simulink model "Modele_LQR_3DOF"  (R2019b)
settings: Solver=VariableStepAuto  StartTime=0.0  StopTime=20  FixedStep=0.1  RelTol=1e-3
undefined symbols (not defined in the file): Amatrix, B, Bmatrix, Fx1, Fx2, Fx3, Fx4, Fx5, Fx6, Fx7, Fx8, Fy1, Fy2, Fy3, Fy4, Fy5, Fy6, Fy7, Fy8, Fz1, Fz2, Fz3, Fz4, Fz5, Fz6, Fz7, Fz8, I_x, I_y, I_z, lx1, lx2, lx3, lx4, lx5, lx6, lx7, lx8, ly1, ly2, ly3, ly4, ly5, ly6, ly7, ly8, lz1, lz2, lz3, lz4, lz5, lz6, lz7, lz8, m, Q, R, W, X0, x_rb ... (+5)
libraries: simulink x12, robotlib x7, dspinverses x1
(part 1 of 2)
settings Model: Creator=ASUQTR  LastModifiedBy=coteba
settings SolverCC: ZeroCrossAlgorithm=Adaptive
settings DebuggingCC: IgnoredZcDiagnostic=none

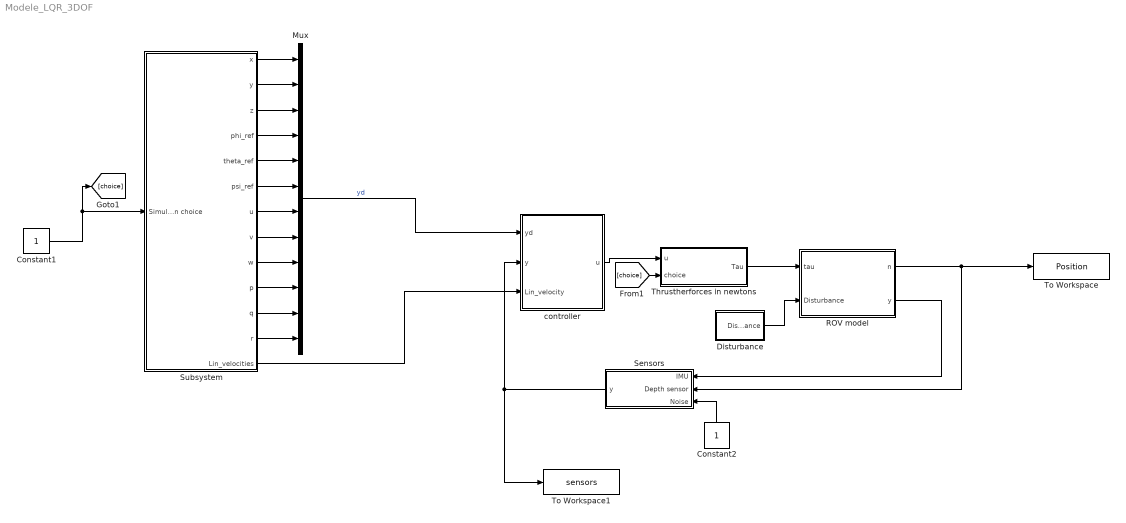
== system Modele_LQR_3DOF ==
  Constant1 : Constant
  Constant2 : Constant
  Disturbance : Subsystem
  Mux : Mux  Inputs=12
  ROV model : Subsystem
  Sensors : Subsystem
  Subsystem : Subsystem
  Thrustherforces in newtons : Subsystem
  To Workspace : ToWorkspace  VariableName=Position  SaveFormat=Structure With Time  SampleTime=-1
  To Workspace1 : ToWorkspace  VariableName=sensors  SaveFormat=Structure With Time  SampleTime=-1
  controller : Subsystem
  wires:
  Mux/1 -> controller/1(yd)  "yd"
  Disturbance/1(Disturbance) -> ROV model/2(Disturbance)
  ROV model/1(n) -> To Workspace/1, Sensors/2(Depth sensor)
  Thrustherforces in newtons/1(Tau) -> ROV model/1(tau)
  controller/1(u) -> Thrustherforces in newtons/1(u)
  Constant1/1 -> [choice], Subsystem/1(Simulation choice)
  Subsystem/13(Lin_velocities) -> controller/3(Lin_velocity)
  [choice] -> Thrustherforces in newtons/2(choice)
  Constant2/1 -> Sensors/3(Noise)
  ROV model/2(y) -> Sensors/1(IMU)
  Subsystem/2("y ") -> Mux/2
  Subsystem/1(x) -> Mux/1
  Subsystem/3("z ") -> Mux/3
  Subsystem/4(phi_ref) -> Mux/4
  Subsystem/5(theta_ref) -> Mux/5
  Subsystem/6(psi_ref) -> Mux/6
  Subsystem/7(u) -> Mux/7
  Subsystem/8(v) -> Mux/8
  Subsystem/9(w) -> Mux/9
  Subsystem/10(p) -> Mux/10
  Subsystem/11(q) -> Mux/11
  Subsystem/12(r) -> Mux/12
  Sensors/1(y) -> To Workspace1/1, controller/2(y)

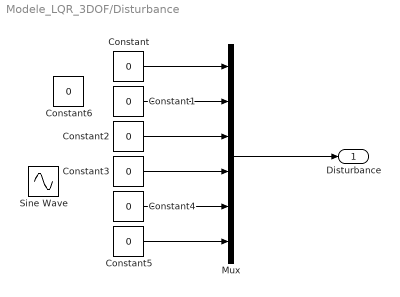
== system Modele_LQR_3DOF/Disturbance ==
  Constant{,1..6} (7 alike) : Constant  Value=0
  Mux : Mux  Inputs=6
  Sine Wave : Sin  Amplitude=0.15  Frequency=10  SampleTime=0
  Disturbance : Outport
  wires:
  Mux/1 -> Disturbance/1
  Constant1/1 -> Mux/2
  Constant2/1 -> Mux/3
  Constant4/1 -> Mux/5
  Constant5/1 -> Mux/6
  Constant/1 -> Mux/1
  Constant3/1 -> Mux/4

== system Modele_LQR_3DOF/ROV model ==
  tau : Inport
  Disturbance : Inport  Port=2
  ROV model : Subsystem
  n : Outport
  y : Outport  Port=2
  wires:
  tau/1 -> ROV model/1(tau)
  Disturbance/1 -> ROV model/2(Disturbance)
  ROV model/2(euler+vitesse_body) -> y/1
  ROV model/1(𝜂) -> n/1

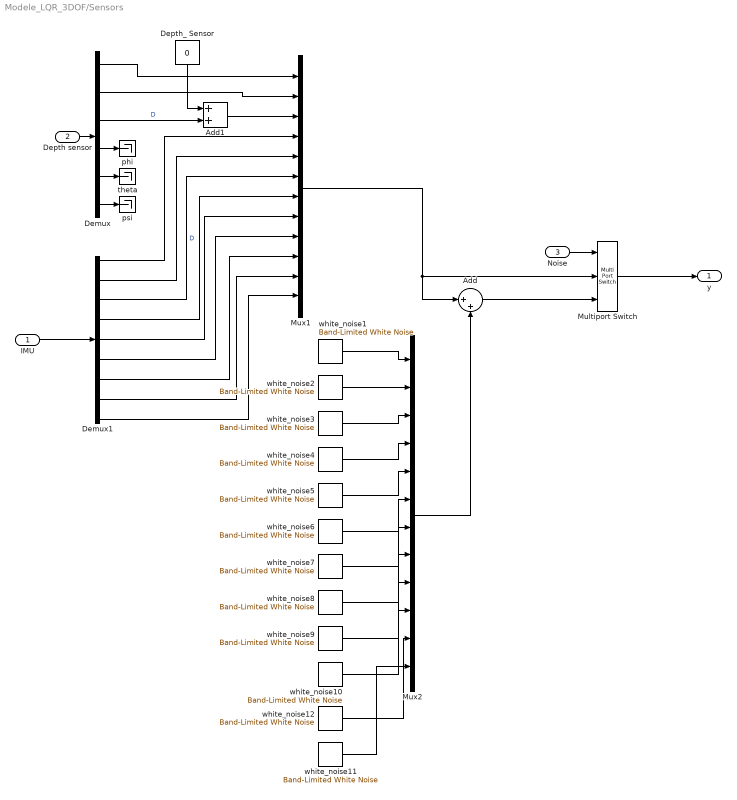
== system Modele_LQR_3DOF/Sensors ==
  IMU : Inport
  Depth sensor : Inport  Port=2
  Noise : Inport  Port=3
  Add : Sum  Inputs=|++
  Add1 : Sum
  Demux : Demux  Outputs=6
  Demux1 : Demux  Outputs=9
  Depth_ Sensor : Constant  Value=0
  Multiport Switch : MultiPortSwitch  Inputs=2
  Mux1 : Mux  Inputs=12
  Mux2 : Mux  Inputs=12
  phi : Terminator
  psi : Terminator
  theta : Terminator
  white_noise1 : simulink/Sources/Band-Limited White Noise  Cov=0.000010  Ts=0.01  seed=[23341]
  white_noise{7..12} (6 alike) : simulink/Sources/Band-Limited White Noise  Cov=0.000010  Ts=0.010000  seed=[8093341]
  white_noise2 : simulink/Sources/Band-Limited White Noise  Cov=0.000010  Ts=0.010000  seed=[23312341]
  white_noise3 : simulink/Sources/Band-Limited White Noise  Cov=0.000010  Ts=0.010000  seed=[2334571]
  white_noise4 : simulink/Sources/Band-Limited White Noise  Cov=0.000010  Ts=0.010000  seed=[21344441]
  white_noise5 : simulink/Sources/Band-Limited White Noise  Cov=0.000010  Ts=0.010000  seed=[3304141]
  white_noise6 : simulink/Sources/Band-Limited White Noise  Cov=0.000010  Ts=0.010000  seed=[903341]
  y : Outport
  wires:
  Multiport Switch/1 -> y/1
  Add/1 -> Multiport Switch/3
  white_noise5/1 -> Mux2/5
  white_noise6/1 -> Mux2/6
  white_noise4/1 -> Mux2/4
  white_noise2/1 -> Mux2/2
  white_noise1/1 -> Mux2/1
  white_noise3/1 -> Mux2/3
  white_noise7/1 -> Mux2/7
  Mux2/1 -> Add/2
  Noise/1 -> Multiport Switch/1
  Mux1/1 -> Multiport Switch/2, Add/1
  white_noise8/1 -> Mux2/8
  white_noise9/1 -> Mux2/9
  white_noise10/1 -> Mux2/10
  Depth sensor/1 -> Demux/1
  Demux/4 -> phi/1
  Demux/5 -> theta/1
  Demux/6 -> psi/1
  Demux/3 -> Add1/2  "D"
  Depth_ Sensor/1 -> Add1/1
  IMU/1 -> Demux1/1
  Add1/1 -> Mux1/3
  Demux/2 -> Mux1/2
  Demux/1 -> Mux1/1
  Demux1/1 -> Mux1/4
  Demux1/2 -> Mux1/5
  Demux1/3 -> Mux1/6  "D"
  Demux1/4 -> Mux1/7
  Demux1/5 -> Mux1/8
  Demux1/6 -> Mux1/9
  Demux1/7 -> Mux1/10
  Demux1/8 -> Mux1/11
  Demux1/9 -> Mux1/12
  white_noise12/1 -> Mux2/11
  white_noise11/1 -> Mux2/12

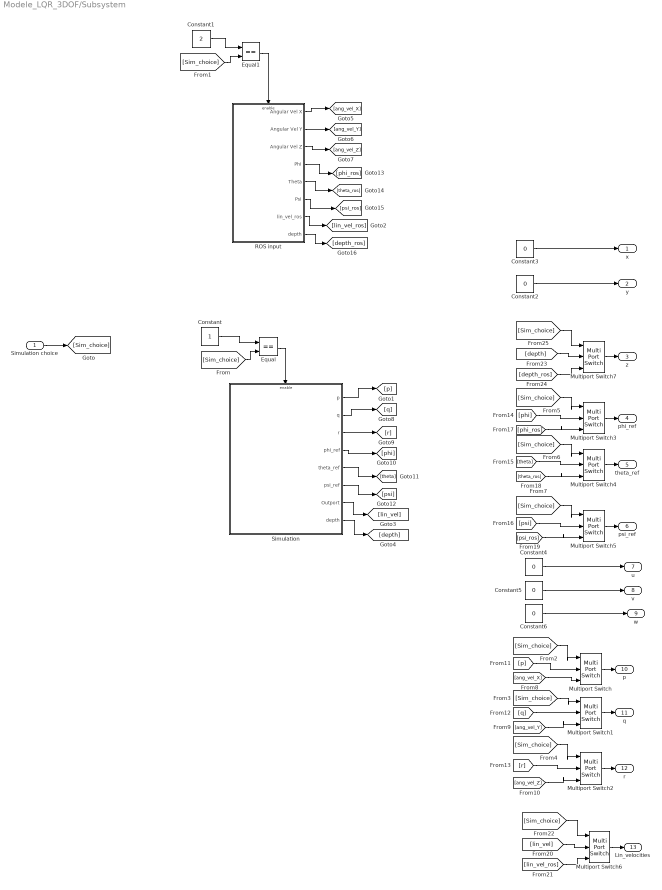
== system Modele_LQR_3DOF/Subsystem ==
  Simulation choice : Inport
  Constant : Constant
  Constant1 : Constant  Value=2
  Constant{2..6} (5 alike) : Constant  Value=0
  Equal : RelationalOperator  Operator===  OutDataTypeStr=boolean  RndMeth=Simplest
  Equal1 : RelationalOperator  Operator===  OutDataTypeStr=boolean  RndMeth=Simplest
  Multiport Switch{,1..7} (8 alike) : MultiPortSwitch  Inputs=2
  ROS input : Subsystem
  Simulation : Subsystem
  x : Outport  VectorParamsAs1DForOutWhenUnconnected=off
  "y " : Outport  Port=2  VectorParamsAs1DForOutWhenUnconnected=off
  "z " : Outport  Port=3  VectorParamsAs1DForOutWhenUnconnected=off
  phi_ref : Outport  Port=4  VectorParamsAs1DForOutWhenUnconnected=off
  theta_ref : Outport  Port=5  VectorParamsAs1DForOutWhenUnconnected=off
  psi_ref : Outport  Port=6  VectorParamsAs1DForOutWhenUnconnected=off
  u : Outport  Port=7  VectorParamsAs1DForOutWhenUnconnected=off
  v : Outport  Port=8  VectorParamsAs1DForOutWhenUnconnected=off
  w : Outport  Port=9  VectorParamsAs1DForOutWhenUnconnected=off
  p : Outport  Port=10  VectorParamsAs1DForOutWhenUnconnected=off
  q : Outport  Port=11  VectorParamsAs1DForOutWhenUnconnected=off
  r : Outport  Port=12  VectorParamsAs1DForOutWhenUnconnected=off
  Lin_velocities : Outport  Port=13  VectorParamsAs1DForOutWhenUnconnected=off
  wires:
  Equal/1 -> Simulation/Enable
  Simulation choice/1 -> [Sim_choice]
  Constant/1 -> Equal/1
  [Sim_choice] -> Equal/2
  Constant1/1 -> Equal1/1
  [Sim_choice] -> Equal1/2
  Equal1/1 -> ROS input/Enable
  Multiport Switch/1 -> p/1
  Multiport Switch1/1 -> q/1
  Multiport Switch2/1 -> r/1
  Multiport Switch3/1 -> phi_ref/1
  Multiport Switch4/1 -> theta_ref/1
  Multiport Switch5/1 -> psi_ref/1
  [Sim_choice] -> Multiport Switch/1
  [Sim_choice] -> Multiport Switch1/1
  [Sim_choice] -> Multiport Switch2/1
  [Sim_choice] -> Multiport Switch3/1
  [Sim_choice] -> Multiport Switch4/1
  [Sim_choice] -> Multiport Switch5/1
  ROS input/1(Angular Vel X) -> [ang_vel_X]
  ROS input/2(Angular Vel Y) -> [ang_vel_Y]
  ROS input/3(Angular Vel Z) -> [ang_vel_Z]
  [ang_vel_X] -> Multiport Switch/3
  [ang_vel_Y] -> Multiport Switch1/3
  [ang_vel_Z] -> Multiport Switch2/3
  Simulation/1(p) -> [p]
  Simulation/2(q) -> [q]
  Simulation/3(r) -> [r]
  Simulation/4(phi_ref) -> [phi]
  Simulation/5(theta_ref) -> [theta]
  Simulation/6(psi_ref) -> [psi]
  [p] -> Multiport Switch/2
  [q] -> Multiport Switch1/2
  [r] -> Multiport Switch2/2
  [phi] -> Multiport Switch3/2
  [theta] -> Multiport Switch4/2
  [psi] -> Multiport Switch5/2
  ROS input/4(Phi) -> [phi_ros]
  ROS input/5(Theta) -> [theta_ros]
  ROS input/6(Psi) -> [psi_ros]
  [phi_ros] -> Multiport Switch3/3
  [theta_ros] -> Multiport Switch4/3
  [psi_ros] -> Multiport Switch5/3
  Simulation/7(Outport) -> [lin_vel]
  [lin_vel_ros] -> Multiport Switch6/3
  [Sim_choice] -> Multiport Switch6/1
  [lin_vel] -> Multiport Switch6/2
  Multiport Switch6/1 -> Lin_velocities/1
  ROS input/7(lin_vel_ros) -> [lin_vel_ros]
  [depth] -> Multiport Switch7/2
  [depth_ros] -> Multiport Switch7/3
  Multiport Switch7/1 -> "z "/1
  [Sim_choice] -> Multiport Switch7/1
  Simulation/8(depth) -> [depth]
  ROS input/8(depth) -> [depth_ros]
  Constant2/1 -> "y "/1
  Constant3/1 -> x/1
  Constant4/1 -> u/1
  Constant5/1 -> v/1
  Constant6/1 -> w/1

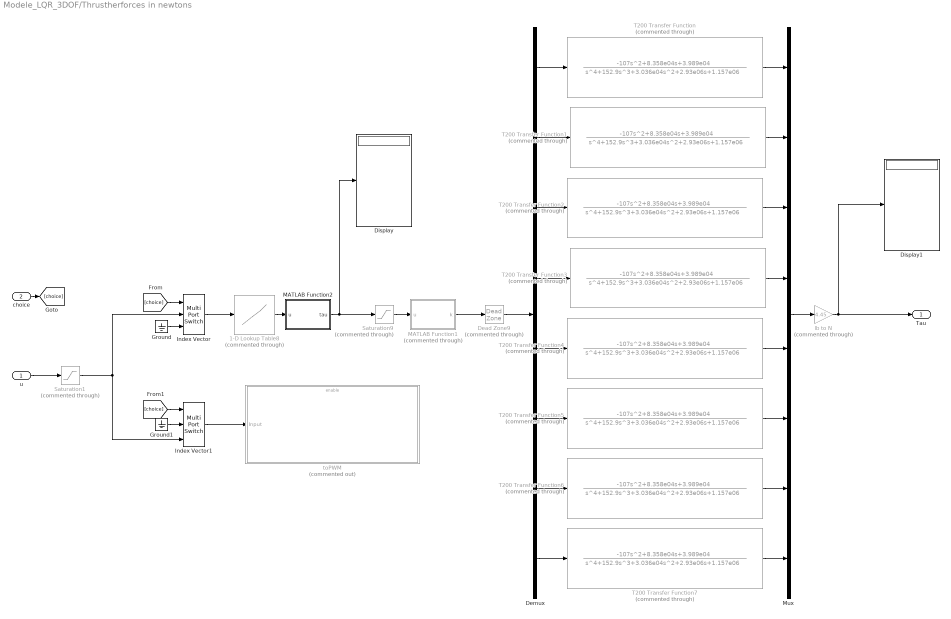
== system Modele_LQR_3DOF/Thrustherforces in newtons ==
  u : Inport
  choice : Inport  Port=2
  1-D Lookup Table8 : Lookup_n-D  Commented=through  NumberOfTableDimensions=1  BreakpointsForDimension1=[-1:0.01:1]  Table=1500 + 400 * ([-1:0.01:1])  InternalRulePriority=Speed  RndMeth=Simplest  InputSameDT=on
  Dead Zone9 : DeadZone  Commented=through  LowerValue=-10  UpperValue=+10  SaturateOnIntegerOverflow=on
  Demux : Demux  Outputs=8
  Display : Display
  Display1 : Display
  Ground : Ground
  Ground1 : Ground
  Index Vector : MultiPortSwitch  DataPortOrder=Specify indices  Inputs=1  DataPortIndices={1,2}
  Index Vector1 : MultiPortSwitch  DataPortOrder=Specify indices  Inputs=2  DataPortIndices={1,2}
  MATLAB Function1 : MATLAB Function  Commented=through  TreatAsAtomicUnit=on
  MATLAB Function2 : MATLAB Function  TreatAsAtomicUnit=on
  Mux : Mux  Inputs=8
  Saturation1 : Saturate  Commented=through  UpperLimit=1  LowerLimit=-1
  Saturation9 : Saturate  Commented=through  UpperLimit=1900  LowerLimit=1100
  T200 Transfer Function{,1..7} (8 alike) : TransferFcn  Commented=through  Numerator="[-107  8.358e04  3.989e04]"  Denominator="[1 152.9  3.036e04  2.93e06  1.157e06]"
  lb to N : Gain  Commented=through  Gain=4.45
  toPWM : Subsystem  Commented=on
  Tau : Outport
  wires:
  u/1 -> Saturation1/1
  Demux/5 -> T200 Transfer Function4/1
  Demux/4 -> T200 Transfer Function3/1
  Demux/2 -> T200 Transfer Function1/1
  1-D Lookup Table8/1 -> MATLAB Function2/1(u)
  Demux/1 -> T200 Transfer Function/1
  Demux/3 -> T200 Transfer Function2/1
  Demux/6 -> T200 Transfer Function5/1
  Demux/7 -> T200 Transfer Function6/1
  Demux/8 -> T200 Transfer Function7/1
  Dead Zone9/1 -> Demux/1
  T200 Transfer Function1/1 -> Mux/2
  T200 Transfer Function3/1 -> Mux/4
  T200 Transfer Function2/1 -> Mux/3
  T200 Transfer Function/1 -> Mux/1
  T200 Transfer Function4/1 -> Mux/5
  T200 Transfer Function5/1 -> Mux/6
  T200 Transfer Function6/1 -> Mux/7
  T200 Transfer Function7/1 -> Mux/8
  Mux/1 -> lb to N/1
  lb to N/1 -> Display1/1, Tau/1
  Index Vector1/1 -> toPWM/1(Input)
  Saturation1/1 -> Index Vector/2, Index Vector1/3
  Ground/1 -> Index Vector/3
  Ground1/1 -> Index Vector1/2
  choice/1 -> [choice]
  [choice] -> Index Vector/1
  [choice] -> Index Vector1/1
  Index Vector/1 -> 1-D Lookup Table8/1
  Saturation9/1 -> MATLAB Function1/1(u)
  MATLAB Function1/1(k) -> Dead Zone9/1
  MATLAB Function2/1(tau) -> Display/1, Saturation9/1

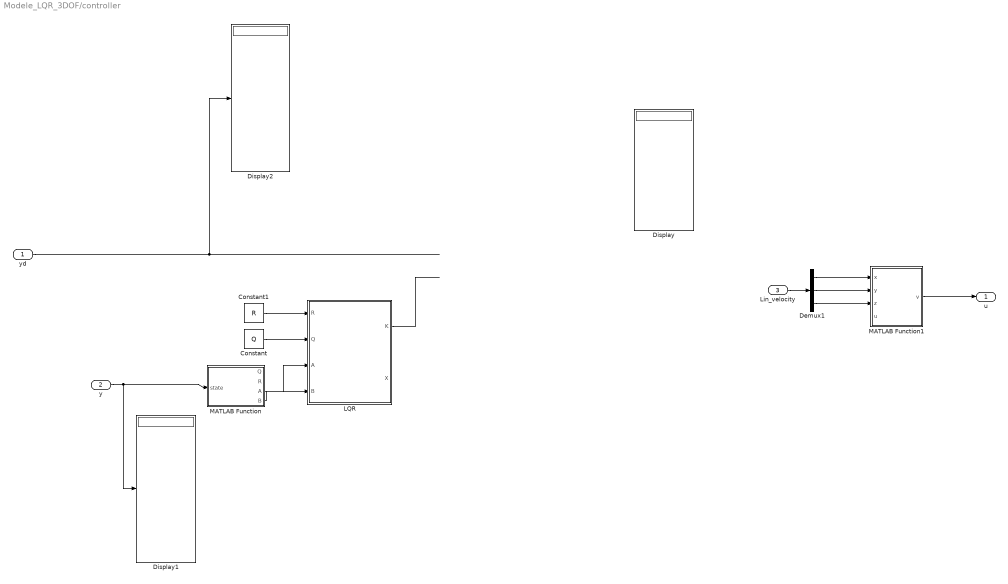
== system Modele_LQR_3DOF/controller ==
  yd : Inport
  y : Inport  Port=2
  Lin_velocity : Inport  Port=3
  Constant : Constant  Value=Q
  Constant1 : Constant  Value=R
  Demux1 : Demux  Outputs=3
  Display : Display
  Display1 : Display
  Display2 : Display
  LQR : Subsystem  Description=|  TreatAsAtomicUnit=on  mask(LQR with Algebric Riccati Equation){A=Amatrix, B=Bmatrix, X0=X0}
      | LQR Block
      | 
      | by Gurkan KAVURAN
      | gurkankavuran@gmail.com
      mask prompts: A "A (System Matrix)"; B "B (System Matrix)"; X0 "Xo (Initial Values of States)"
      mask help:
      | It is easy to optimize Q and R matrices with online process.
      | Please see the help file to define the block parameters.
      mask Help:
      | Parameters Example:
      | 
      | Q = diag([500 1 1 0 1 1] );
      | R = 1*diag([0.01 0.01 0.01 0.01]);
      | X0=[0 0 0 0 0 0;0 0 0 0 0 0;0 0 0 0 0 0;0 0 0 0 0 0;0 0 0 0 0 0;0 0 0 0 0 0];
      | 
      | "Matrix multiply" block is recommended to use in state feedback control mechanism.
      | 
      | 
      | http://www.gurkankavuran.com
      mask Display:
      | disp('LQR')
      | port_label('input', 1, 'R')
      | port_label('input', 2, 'Q')
      | port_label('output', 1, 'K')
      | port_label('output', 2, 'X')
  MATLAB Function : MATLAB Function  TreatAsAtomicUnit=on
  MATLAB Function1 : MATLAB Function  TreatAsAtomicUnit=on
  u : Outport
  wires:
  Constant1/1 -> LQR/1(R)
  Constant/1 -> LQR/2(Q)
  LQR/1(K) -> ?
  ? -> MATLAB Function1/4(u), Display/1
  Lin_velocity/1 -> Demux1/1
  yd/1 -> Display2/1
  MATLAB Function1/1(v) -> u/1
  Demux1/2 -> MATLAB Function1/2(y)
  Demux1/1 -> MATLAB Function1/1(x)
  Demux1/3 -> MATLAB Function1/3(z)
  MATLAB Function/3(A) -> LQR/3(A)
  MATLAB Function/4(B) -> LQR/4("B ")
  y/1 -> Display1/1, MATLAB Function/1(state)

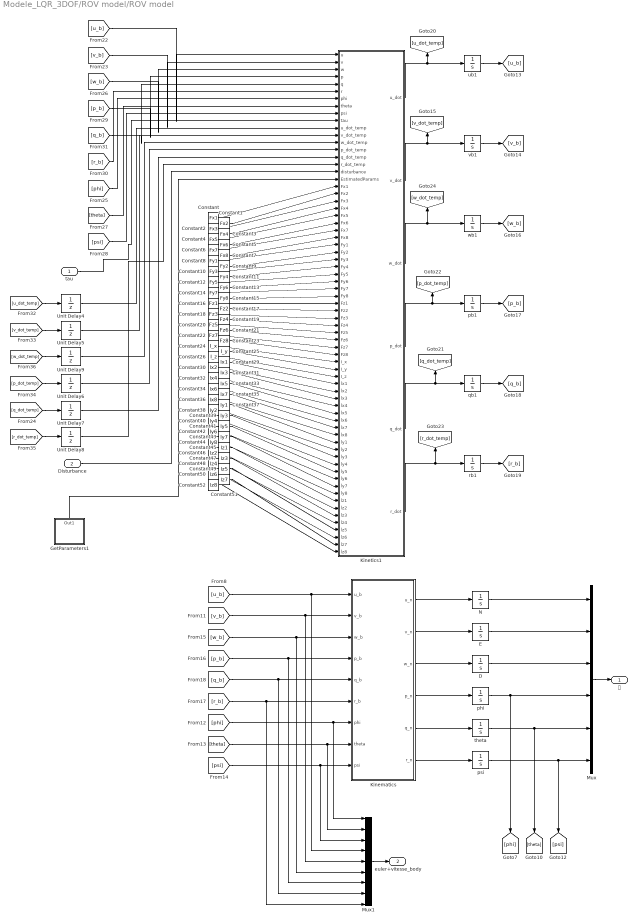
== system Modele_LQR_3DOF/ROV model/ROV model ==
  tau : Inport
  Disturbance : Inport  Port=2
  Constant : Constant  Value=Fx1
  Constant1 : Constant  Value=Fx2
  Constant10 : Constant  Value=Fy3
  Constant11 : Constant  Value=Fy4
  Constant12 : Constant  Value=Fy5
  Constant13 : Constant  Value=Fy6
  Constant14 : Constant  Value=Fy7
  Constant15 : Constant  Value=Fy8
  Constant16 : Constant  Value=Fz1
  Constant17 : Constant  Value=Fz2
  Constant18 : Constant  Value=Fz3
  Constant19 : Constant  Value=Fz4
  Constant2 : Constant  Value=Fx3
  Constant20 : Constant  Value=Fz5
  Constant21 : Constant  Value=Fz6
  Constant22 : Constant  Value=Fz7
  Constant23 : Constant  Value=Fz8
  Constant24 : Constant  Value=I_x
  Constant25 : Constant  Value=I_y
  Constant26 : Constant  Value=I_z
  Constant29 : Constant  Value=lx1
  Constant3 : Constant  Value=Fx4
  Constant30 : Constant  Value=lx2
  Constant31 : Constant  Value=lx3
  Constant32 : Constant  Value=lx4
  Constant33 : Constant  Value=lx5
  Constant34 : Constant  Value=lx6
  Constant35 : Constant  Value=lx7
  Constant36 : Constant  Value=lx8
  Constant37 : Constant  Value=ly1
  Constant38 : Constant  Value=ly2
  Constant39 : Constant  Value=ly3
  Constant4 : Constant  Value=Fx5
  Constant40 : Constant  Value=ly4
  Constant41 : Constant  Value=ly5
  Constant42 : Constant  Value=ly6
  Constant43 : Constant  Value=ly7
  Constant44 : Constant  Value=ly8
  Constant45 : Constant  Value=lz1
  Constant46 : Constant  Value=lz2
  Constant47 : Constant  Value=lz3
  Constant48 : Constant  Value=lz4
  Constant49 : Constant  Value=lz5
  Constant5 : Constant  Value=Fx6
  Constant50 : Constant  Value=lz6
  Constant51 : Constant  Value=lz7
  Constant52 : Constant  Value=lz8
  Constant6 : Constant  Value=Fx7
  Constant7 : Constant  Value=Fx8
  Constant8 : Constant  Value=Fy1
  Constant9 : Constant  Value=Fy2
  D : Integrator  InitialCondition=0.0000001  ContinuousStateAttributes='phi'
  E : Integrator  InitialCondition=0.0000001  ContinuousStateAttributes='phi'
  GetParameters1 : Subsystem
  Kinematics : MATLAB Function  TreatAsAtomicUnit=on
  Kinetics1 : MATLAB Function  TreatAsAtomicUnit=on
  Mux : Mux  Inputs=6
  Mux1 : Mux  Inputs=9
  N : Integrator  InitialCondition=0.0000001  ContinuousStateAttributes='phi'
  Unit Delay{4..9} (6 alike) : UnitDelay  SampleTime=0.01  HasFrameUpgradeWarning=on
  pb1 : Integrator  InitialCondition=0.0000001
  phi : Integrator  InitialCondition=0.0000001  ContinuousStateAttributes='phi'
  psi : Integrator  InitialCondition=0.0000001  ContinuousStateAttributes='psi'
  qb1 : Integrator  InitialCondition=0.0000001
  rb1 : Integrator  InitialCondition=0.0000001
  theta : Integrator  InitialCondition=0.0000001  ContinuousStateAttributes='theta'
  ub1 : Integrator  InitialCondition=0.0000001
  vb1 : Integrator  InitialCondition=0.0000001
  wb1 : Integrator  InitialCondition=0.0000001
  𝜂 : Outport
  euler+vitesse_body : Outport  Port=2
  wires:
  Unit Delay9/1 -> Kinetics1/13(w_dot_temp)
  tau/1 -> Kinetics1/10(tau)
  [phi] -> Kinetics1/7(phi)
  Kinetics1/4(p_dot) -> [p_dot_temp], pb1/1
  [w_dot_temp] -> Unit Delay9/1
  Kinetics1/2(v_dot) -> [v_dot_temp], vb1/1
  [r_b] -> Kinetics1/6(r)
  Kinetics1/6(r_dot) -> rb1/1, [r_dot_temp]
  Unit Delay8/1 -> Kinetics1/16(r_dot_temp)
  [u_b] -> Kinetics1/1(u)
  Unit Delay7/1 -> Kinetics1/15(q_dot_temp)
  rb1/1 -> [r_b]
  Unit Delay6/1 -> Kinetics1/14(p_dot_temp)
  [q_b] -> Kinetics1/5(q)
  [r_dot_temp] -> Unit Delay8/1
  [psi] -> Kinetics1/9(psi)
  [p_dot_temp] -> Unit Delay6/1
  [q_dot_temp] -> Unit Delay7/1
  [p_b] -> Kinetics1/4(p)
  Disturbance/1 -> Kinetics1/17(disturbance)
  Kinetics1/1(u_dot) -> [u_dot_temp], ub1/1
  Unit Delay5/1 -> Kinetics1/12(v_dot_temp)
  [theta] -> Kinetics1/8(theta)
  Kinetics1/5(q_dot) -> qb1/1, [q_dot_temp]
  [v_b] -> Kinetics1/2(v)
  GetParameters1/1(Out1) -> Kinetics1/18(EstimatedParams)
  [w_b] -> Kinetics1/3(w)
  pb1/1 -> [p_b]
  [v_dot_temp] -> Unit Delay5/1
  qb1/1 -> [q_b]
  vb1/1 -> [v_b]
  ub1/1 -> [u_b]
  wb1/1 -> [w_b]
  Kinetics1/3(w_dot) -> [w_dot_temp], wb1/1
  [u_dot_temp] -> Unit Delay4/1
  Unit Delay4/1 -> Kinetics1/11(u_dot_temp)
  [r_b] -> Mux1/9, Kinematics/6(r_b)
  [w_b] -> Mux1/6, Kinematics/3(w_b)
  Kinematics/4(p_n) -> phi/1
  Mux1/1 -> euler+vitesse_body/1
  phi/1 -> Mux/4, [phi]
  Kinematics/5(q_n) -> theta/1
  psi/1 -> Mux/6, [psi]
  [phi] -> Mux1/1, Kinematics/7(phi)
  Kinematics/1(u_n) -> N/1
  [theta] -> Mux1/2, Kinematics/8(theta)
  Kinematics/6(r_n) -> psi/1
  Kinematics/3(w_n) -> D/1
  D/1 -> Mux/3
  E/1 -> Mux/2
  [q_b] -> Mux1/8, Kinematics/5(q_b)
  N/1 -> Mux/1
  [u_b] -> Mux1/4, Kinematics/1(u_b)
  [v_b] -> Mux1/5, Kinematics/2(v_b)
  theta/1 -> Mux/5, [theta]
  [p_b] -> Mux1/7, Kinematics/4(p_b)
  [psi] -> Mux1/3, Kinematics/9(psi)
  Kinematics/2(v_n) -> E/1
  Mux/1 -> 𝜂/1
  Constant/1 -> Kinetics1/19(Fx1)
  Constant1/1 -> Kinetics1/20(Fx2)
  Constant2/1 -> Kinetics1/21(Fx3)
  Constant3/1 -> Kinetics1/22(Fx4)
  Constant4/1 -> Kinetics1/23(Fx5)
  Constant5/1 -> Kinetics1/24(Fx6)
  Constant6/1 -> Kinetics1/25(Fx7)
  Constant7/1 -> Kinetics1/26(Fx8)
  Constant8/1 -> Kinetics1/27(Fy1)
  Constant9/1 -> Kinetics1/28(Fy2)
  Constant10/1 -> Kinetics1/29(Fy3)
  Constant11/1 -> Kinetics1/30(Fy4)
  Constant12/1 -> Kinetics1/31(Fy5)
  Constant13/1 -> Kinetics1/32(Fy6)
  Constant14/1 -> Kinetics1/33(Fy7)
  Constant15/1 -> Kinetics1/34(Fy8)
  Constant16/1 -> Kinetics1/35(Fz1)
  Constant17/1 -> Kinetics1/36(Fz2)
  Constant18/1 -> Kinetics1/37(Fz3)
  Constant19/1 -> Kinetics1/38(Fz4)
  Constant20/1 -> Kinetics1/39(Fz5)
  Constant21/1 -> Kinetics1/40(Fz6)
  Constant22/1 -> Kinetics1/41(Fz7)
  Constant23/1 -> Kinetics1/42(Fz8)
  Constant24/1 -> Kinetics1/43(I_x)
  Constant25/1 -> Kinetics1/44(I_y)
  Constant26/1 -> Kinetics1/45(I_z)
  Constant34/1 -> Kinetics1/51(lx6)
  Constant33/1 -> Kinetics1/50(lx5)
  Constant35/1 -> Kinetics1/52(lx7)
  Constant31/1 -> Kinetics1/48(lx3)
  Constant32/1 -> Kinetics1/49(lx4)
  Constant30/1 -> Kinetics1/47(lx2)
  Constant29/1 -> Kinetics1/46(lx1)
  Constant36/1 -> Kinetics1/53(lx8)
  Constant38/1 -> Kinetics1/55(ly2)
  Constant37/1 -> Kinetics1/54(ly1)
  Constant44/1 -> Kinetics1/61(ly8)
  Constant43/1 -> Kinetics1/60(ly7)
  Constant45/1 -> Kinetics1/62(lz1)
  Constant41/1 -> Kinetics1/58(ly5)
  Constant42/1 -> Kinetics1/59(ly6)
  Constant40/1 -> Kinetics1/57(ly4)
  Constant39/1 -> Kinetics1/56(ly3)
  Constant46/1 -> Kinetics1/63(lz2)
  Constant48/1 -> Kinetics1/65(lz4)
  Constant47/1 -> Kinetics1/64(lz3)
  Constant51/1 -> Kinetics1/68(lz7)
  Constant52/1 -> Kinetics1/69(lz8)
  Constant50/1 -> Kinetics1/67(lz6)
  Constant49/1 -> Kinetics1/66(lz5)

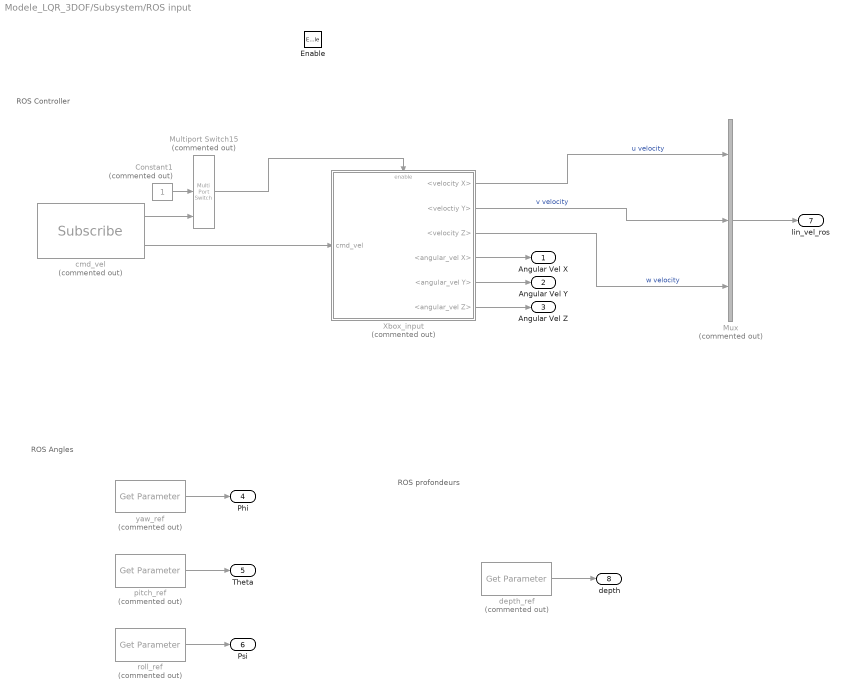
== system Modele_LQR_3DOF/Subsystem/ROS input ==
  note: ROS
      | Angles
  note: ROS
      | Controller
  note: ROS
      | profondeurs
  Enable : EnablePort
  Constant1 : Constant  Commented=on
  Multiport Switch15 : MultiPortSwitch  Commented=on  Inputs=2
  Mux : Mux  Commented=on  Inputs=3
  Xbox_input : Subsystem  Commented=on
  cmd_vel : robotlib/Subscribe  Commented=on  topicSource=Select from ROS network  topic=/cmd_vel  messageType=geometry_msgs/Twist  sampleTime=-1  messageQueueLength=10
      link override SourceBlock: ROSTopic=/cmd_vel  ROSMessageType=geometry_msgs/Twist  SLBusName=SL_Bus_simplified_modele_geometry_msgs_Twist  ModelName=simplified_modele  BlockId=Sub_simplified_modele_856
      settings: SourceProductBaseCode=RO
  depth_ref : robotlib/Get Parameter  Commented=on  ParameterSource=Select from ROS network  ParameterName=/MatlabController/yaw_ref  ParameterType=double  ParameterMaxArrayLength=16  ParameterInitialValue=0  SampleTime=-1  ShowErrorCodeOutput=off  ModelName=simplified_modele  BlockId=ParamGet_simplified_modele_974
      settings: SourceProductName=ROS Toolbox  SourceProductBaseCode=RR
  pitch_ref : robotlib/Get Parameter  Commented=on  ParameterSource=Select from ROS network  ParameterName=/MatlabController/pitch_ref  ParameterType=double  ParameterMaxArrayLength=16  ParameterInitialValue=0  SampleTime=-1  ShowErrorCodeOutput=off  ModelName=simplified_modele  BlockId=ParamGet_simplified_modele_975
      settings: SourceProductName=ROS Toolbox  SourceProductBaseCode=RR
  roll_ref : robotlib/Get Parameter  Commented=on  ParameterSource=Select from ROS network  ParameterName=/MatlabController/roll_ref  ParameterType=double  ParameterMaxArrayLength=16  ParameterInitialValue=0  SampleTime=-1  ShowErrorCodeOutput=off  ModelName=simplified_modele  BlockId=ParamGet_simplified_modele_976
      settings: SourceProductName=ROS Toolbox  SourceProductBaseCode=RR
  yaw_ref : robotlib/Get Parameter  Commented=on  ParameterSource=Select from ROS network  ParameterName=/MatlabController/yaw_ref  ParameterType=double  ParameterMaxArrayLength=16  ParameterInitialValue=0  SampleTime=-1  ShowErrorCodeOutput=off  ModelName=simplified_modele  BlockId=ParamGet_simplified_modele_974
      settings: SourceProductName=ROS Toolbox  SourceProductBaseCode=RR
  Angular Vel X : Outport
  Angular Vel Y : Outport  Port=2
  Angular Vel Z : Outport  Port=3
  Phi : Outport  Port=4
  Theta : Outport  Port=5
  Psi : Outport  Port=6
  lin_vel_ros : Outport  Port=7
  depth : Outport  Port=8
  wires:
  Xbox_input/6("<angular_vel Z> ") -> Angular Vel Z/1
  Multiport Switch15/1 -> Xbox_input/Enable
  Xbox_input/5(<angular_vel Y>) -> Angular Vel Y/1
  cmd_vel/2 -> Xbox_input/1(cmd_vel)
  cmd_vel/1 -> Multiport Switch15/3
  Xbox_input/4(<angular_vel X>) -> Angular Vel X/1
  Constant1/1 -> Multiport Switch15/2
  yaw_ref/1 -> Phi/1
  pitch_ref/1 -> Theta/1
  roll_ref/1 -> Psi/1
  Mux/1 -> lin_vel_ros/1
  Xbox_input/3(<velocity Z>) -> Mux/3  "w velocity"
  Xbox_input/2(<veloctiy Y>) -> Mux/2  "v velocity"
  Xbox_input/1(<velocity X>) -> Mux/1  "u velocity"
  depth_ref/1 -> depth/1

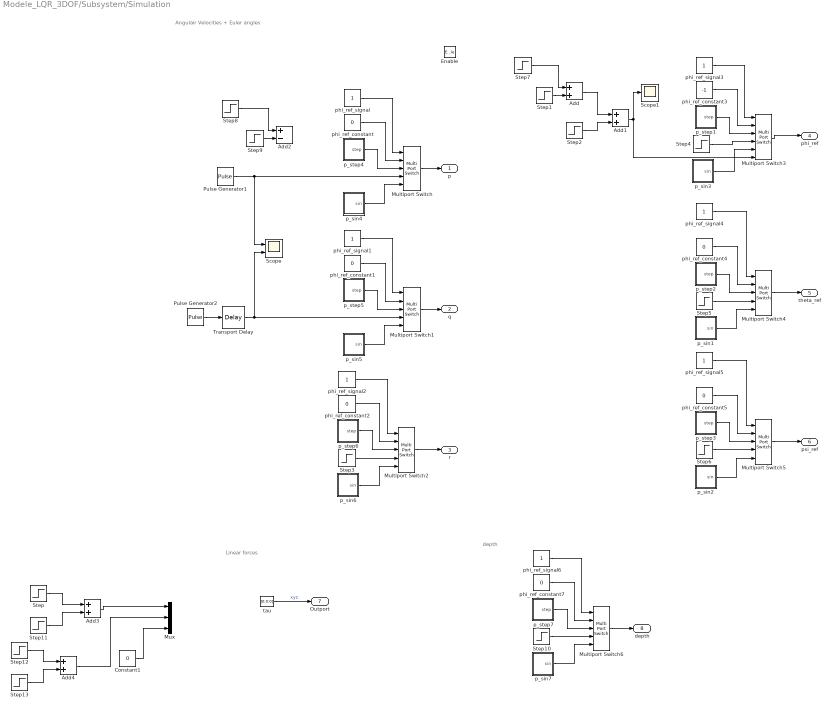
== system Modele_LQR_3DOF/Subsystem/Simulation ==
  note: Linear
      | forces
  note: Angulair
      | Velocities
      | +
      | Euler
      | angles
  note: depth
  Enable : EnablePort
  Add{,1,3..4} (4 alike) : Sum
  Add2 : Sum  Inputs=+-
  Constant1 : Constant  Value=0
  Multiport Switch{,1..2,4..6} (6 alike) : MultiPortSwitch  Inputs=4
  Multiport Switch3 : MultiPortSwitch  Inputs=5
  Mux : Mux  Inputs=3
  Pulse Generator1 : DiscretePulseGenerator  PulseType=Time based  Period=50  PulseWidth=50
  Pulse Generator2 : DiscretePulseGenerator  PulseType=Time based  Period=50  PulseWidth=50
  Scope : Scope  NumInputPorts=2
  Scope1 : Scope
  Step : Step  After=40  SampleTime=0
  Step1 : Step  Time=20  After=1.57  SampleTime=0
  Step10 : Step  After=-5  SampleTime=0
  Step11 : Step  Time=20  After=-40  SampleTime=0
  Step12 : Step  Time=25  After=40  SampleTime=0
  Step13 : Step  Time=45  After=-40  SampleTime=0
  Step2 : Step  Time=32  After=1.57  SampleTime=0
  Step3 : Step  SampleTime=0
  Step4 : Step  Time=20  After=1.57  SampleTime=0
  Step5 : Step  After=1.57  SampleTime=0
  Step6 : Step  After=3  SampleTime=0
  Step7 : Step  Time=5  After=1.57  SampleTime=0
  Step8 : Step  Time=0  After=5  SampleTime=0
  Step9 : Step  Time=0.5  After=2  SampleTime=0
  Transport Delay : TransportDelay  DelayTime=12.5
  p_sin1 : Subsystem
  p_sin2 : Subsystem
  p_sin3 : Subsystem
  p_sin4 : Subsystem
  p_sin5 : Subsystem
  p_sin6 : Subsystem
  p_sin7 : Subsystem
  p_step1 : Subsystem
  p_step2 : Subsystem
  p_step3 : Subsystem
  p_step4 : Subsystem
  p_step5 : Subsystem
  p_step6 : Subsystem
  p_step7 : Subsystem
  phi_ref_constant{,1..2,4..5,7} (6 alike) : Constant  Value=0
  phi_ref_constant3 : Constant  Value=-1
  phi_ref_signal{,1..6} (7 alike) : Constant
  "tau " : Constant  Value=[0;0;0]
  p : Outport  VectorParamsAs1DForOutWhenUnconnected=off
  q : Outport  Port=2  VectorParamsAs1DForOutWhenUnconnected=off
  r : Outport  Port=3  VectorParamsAs1DForOutWhenUnconnected=off
  phi_ref : Outport  Port=4  VectorParamsAs1DForOutWhenUnconnected=off
  theta_ref : Outport  Port=5  VectorParamsAs1DForOutWhenUnconnected=off
  psi_ref : Outport  Port=6  VectorParamsAs1DForOutWhenUnconnected=off
  Outport : Outport  Port=7
  depth : Outport  Port=8
  wires:
  Multiport Switch2/1 -> r/1
  Step3/1 -> Multiport Switch2/4
  phi_ref_signal5/1 -> Multiport Switch5/1
  Add1/1 -> Multiport Switch3/6, Scope1/1
  Step9/1 -> Add2/2
  phi_ref_constant4/1 -> Multiport Switch4/2
  Multiport Switch/1 -> p/1
  Step7/1 -> Add/1
  Pulse Generator1/1 -> Multiport Switch/4, Scope/1
  phi_ref_constant2/1 -> Multiport Switch2/2
  phi_ref_constant5/1 -> Multiport Switch5/2
  p_sin1/1(sin) -> Multiport Switch4/5
  p_sin2/1(sin) -> Multiport Switch5/5
  p_step3/1(step) -> Multiport Switch5/3
  Add/1 -> Add1/1
  Step5/1 -> Multiport Switch4/4
  Pulse Generator2/1 -> Transport Delay/1
  Step1/1 -> Add/2
  phi_ref_signal4/1 -> Multiport Switch4/1
  Multiport Switch3/1 -> phi_ref/1
  p_step1/1(step) -> Multiport Switch3/3
  Step6/1 -> Multiport Switch5/4
  Multiport Switch4/1 -> theta_ref/1
  Transport Delay/1 -> Multiport Switch1/4, Scope/2
  phi_ref_constant3/1 -> Multiport Switch3/2
  Step8/1 -> Add2/1
  p_step2/1(step) -> Multiport Switch4/3
  Multiport Switch5/1 -> psi_ref/1
  phi_ref_signal3/1 -> Multiport Switch3/1
  phi_ref_signal1/1 -> Multiport Switch1/1
  p_sin3/1(sin) -> Multiport Switch3/5
  p_sin6/1(sin) -> Multiport Switch2/5
  p_step5/1(step) -> Multiport Switch1/3
  phi_ref_constant/1 -> Multiport Switch/2
  phi_ref_signal/1 -> Multiport Switch/1
  p_sin5/1(sin) -> Multiport Switch1/5
  phi_ref_signal2/1 -> Multiport Switch2/1
  phi_ref_constant1/1 -> Multiport Switch1/2
  p_step6/1(step) -> Multiport Switch2/3
  p_sin4/1(sin) -> Multiport Switch/5
  Multiport Switch1/1 -> q/1
  p_step4/1(step) -> Multiport Switch/3
  Step2/1 -> Add1/2
  Step10/1 -> Multiport Switch6/4
  p_step7/1(step) -> Multiport Switch6/3
  phi_ref_signal6/1 -> Multiport Switch6/1
  phi_ref_constant7/1 -> Multiport Switch6/2
  Multiport Switch6/1 -> depth/1
  p_sin7/1(sin) -> Multiport Switch6/5
  Step/1 -> Add3/1
  Step11/1 -> Add3/2
  Constant1/1 -> Mux/3
  Add4/1 -> Mux/2
  Add3/1 -> Mux/1
  Step4/1 -> Multiport Switch3/4
  Step12/1 -> Add4/1
  Step13/1 -> Add4/2
  "tau "/1 -> Outport/1  "xyz"

== system Modele_LQR_3DOF/Thrustherforces in newtons/toPWM ==
  note: Generates a PWM signal control message to
      | the arduino.
      | ToDo:
      | Verify that messages are sent and
      | Expects input in -1 to 1 range.
      | Will output is in correct range and that
  Input : Inport
  Enable : EnablePort
  "Actuator message " : robotlib/Blank Message  messageClass=Message  entityType=geometry_msgs/Point  messageType=geometry_msgs/Point  SampleTime=-1
      settings: SourceProductBaseCode=RO
  Data Type Conversion : DataTypeConversion  OutDataTypeStr=single  LockScale=on
  MATLAB Function : MATLAB Function  TreatAsAtomicUnit=on
  Publish : robotlib/Publish  topicSource=Select from ROS network  topic=/motors  messageType=asuqtr_actuator_node/ActuatorThrottle  messageQueueLength=1
      settings: SourceProductBaseCode=RO
  wires:
  MATLAB Function/1(msg) -> Publish/1
  Input/1 -> Data Type Conversion/1
  Data Type Conversion/1 -> MATLAB Function/2(data)
  "Actuator message "/1 -> MATLAB Function/1(blankMessage)

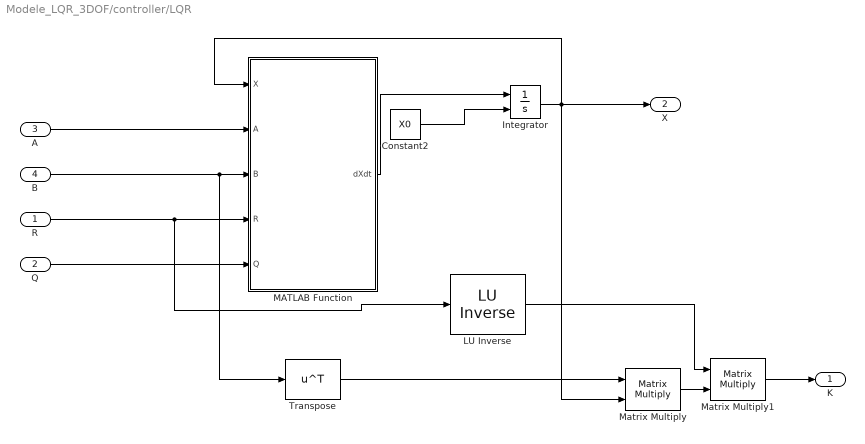
== system Modele_LQR_3DOF/controller/LQR ==
  R : Inport
  Q : Inport  Port=2
  A : Inport  Port=3
  "B " : Inport  Port=4
  " LU Inverse" : dspinverses/ LU Inverse
      settings: SourceProductName=DSP System Toolbox
  Constant2 : Constant  Value=X0
  Integrator : Integrator  InitialConditionSource=external  InitialCondition=[1 1 1 1 1 1 1 1 1 1 1 1 1 1 1 1 1 1 1 1 1 1 1 1 1 1 1 1 1 1 1 1 1 1 1 1]
  MATLAB Function : MATLAB Function  TreatAsAtomicUnit=on
  Matrix Multiply : Product  Multiplication=Matrix(*)
  Matrix Multiply1 : Product  Multiplication=Matrix(*)
  Transpose : Math  Operator=transpose  SignedPower=off  SaturateOnIntegerOverflow=on
  K : Outport
  X : Outport  Port=2
  wires:
  Matrix Multiply1/1 -> K/1
  A/1 -> MATLAB Function/2(A)
  "B "/1 -> Transpose/1, MATLAB Function/3(B)
  " LU Inverse"/1 -> Matrix Multiply1/1
  Constant2/1 -> Integrator/2
  Matrix Multiply/1 -> Matrix Multiply1/2
  Transpose/1 -> Matrix Multiply/1
  MATLAB Function/1(dXdt) -> Integrator/1
  Integrator/1 -> X/1, Matrix Multiply/2, MATLAB Function/1(X)
  Q/1 -> MATLAB Function/5(Q)
  R/1 -> " LU Inverse"/1, MATLAB Function/4(R)

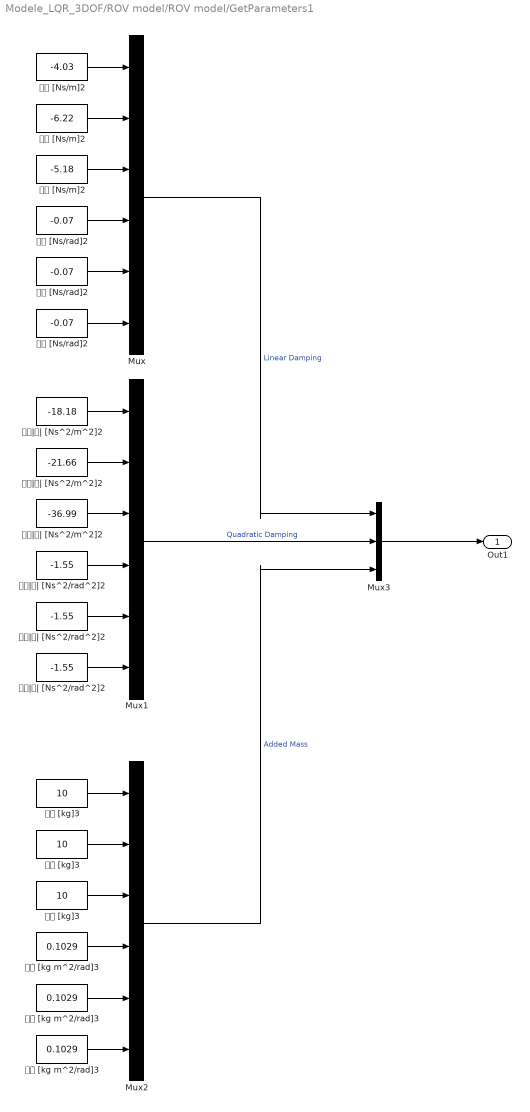
== system Modele_LQR_3DOF/ROV model/ROV model/GetParameters1 ==
  Mux : Mux  Inputs=6
  Mux1 : Mux  Inputs=6
  Mux2 : Mux  Inputs=6
  Mux3 : Mux  Inputs=3
  𝐾𝑝 [Ns/rad]2 : Constant  Value=-0.07
  𝐾𝑝|𝑝| [Ns^2/rad^2]2 : Constant  Value=-1.55
  𝐾𝑝̇ [kg m^2/rad]3 : Constant  Value=0.1029
  𝑀𝑞 [Ns/rad]2 : Constant  Value=-0.07
  𝑀𝑞|𝑞| [Ns^2/rad^2]2 : Constant  Value=-1.55
  𝑀𝑞̇ [kg m^2/rad]3 : Constant  Value=0.1029
  𝑁𝑟 [Ns/rad]2 : Constant  Value=-0.07
  𝑁𝑟|𝑟| [Ns^2/rad^2]2 : Constant  Value=-1.55
  𝑁𝑟̇ [kg m^2/rad]3 : Constant  Value=0.1029
  𝑋𝑢 [Ns/m]2 : Constant  Value=-4.03
  𝑋𝑢|𝑢| [Ns^2/m^2]2 : Constant  Value=-18.18
  𝑋𝑢̇ [kg]3 : Constant  Value=10
  𝑌𝑣 [Ns/m]2 : Constant  Value=-6.22
  𝑌𝑣|𝑣| [Ns^2/m^2]2 : Constant  Value=-21.66
  𝑌𝑣̇ [kg]3 : Constant  Value=10
  𝑍𝑤 [Ns/m]2 : Constant  Value=-5.18
  𝑍𝑤|𝑤| [Ns^2/m^2]2 : Constant  Value=-36.99
  𝑍𝑤̇ [kg]3 : Constant  Value=10
  Out1 : Outport  VectorParamsAs1DForOutWhenUnconnected=off
  wires:
  𝑁𝑟 [Ns/rad]2/1 -> Mux/6
  Mux/1 -> Mux3/1  "Linear Damping"
  𝐾𝑝 [Ns/rad]2/1 -> Mux/4
  𝑀𝑞 [Ns/rad]2/1 -> Mux/5
  𝑍𝑤 [Ns/m]2/1 -> Mux/3
  𝑌𝑣 [Ns/m]2/1 -> Mux/2
  𝑋𝑢 [Ns/m]2/1 -> Mux/1
  𝑌𝑣|𝑣| [Ns^2/m^2]2/1 -> Mux1/2
  𝑍𝑤|𝑤| [Ns^2/m^2]2/1 -> Mux1/3
  𝑋𝑢|𝑢| [Ns^2/m^2]2/1 -> Mux1/1
  Mux1/1 -> Mux3/2  "Quadratic Damping"
  𝑀𝑞|𝑞| [Ns^2/rad^2]2/1 -> Mux1/5
  𝑁𝑟|𝑟| [Ns^2/rad^2]2/1 -> Mux1/6
  𝐾𝑝|𝑝| [Ns^2/rad^2]2/1 -> Mux1/4
  𝐾𝑝̇ [kg m^2/rad]3/1 -> Mux2/4
  Mux2/1 -> Mux3/3  "Added Mass"
  𝑀𝑞̇ [kg m^2/rad]3/1 -> Mux2/5
  𝑋𝑢̇ [kg]3/1 -> Mux2/1
  𝑁𝑟̇ [kg m^2/rad]3/1 -> Mux2/6
  𝑍𝑤̇ [kg]3/1 -> Mux2/3
  𝑌𝑣̇ [kg]3/1 -> Mux2/2
  Mux3/1 -> Out1/1

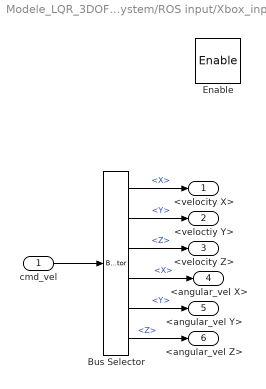
== system Modele_LQR_3DOF/Subsystem/ROS input/Xbox_input ==
  cmd_vel : Inport
  Enable : EnablePort
  Bus Selector : BusSelector  OutputSignals=Linear.X,Linear.Y,Linear.Z,Angular.X,Angular.Y,Angular.Z
  <velocity X> : Outport  VectorParamsAs1DForOutWhenUnconnected=off
  <veloctiy Y> : Outport  Port=2  VectorParamsAs1DForOutWhenUnconnected=off
  <velocity Z> : Outport  Port=3  VectorParamsAs1DForOutWhenUnconnected=off
  <angular_vel X> : Outport  Port=4  VectorParamsAs1DForOutWhenUnconnected=off
  <angular_vel Y> : Outport  Port=5  VectorParamsAs1DForOutWhenUnconnected=off
  "<angular_vel Z> " : Outport  Port=6  VectorParamsAs1DForOutWhenUnconnected=off
  wires:
  cmd_vel/1 -> Bus Selector/1
  Bus Selector/2 -> <veloctiy Y>/1  "<Y>"
  Bus Selector/1 -> <velocity X>/1  "<X>"
  Bus Selector/5 -> <angular_vel Y>/1  "<Y>"
  Bus Selector/3 -> <velocity Z>/1  "<Z>"
  Bus Selector/6 -> "<angular_vel Z> "/1  "<Z>"
  Bus Selector/4 -> <angular_vel X>/1  "<X>"

== system Modele_LQR_3DOF/Subsystem/Simulation/p_sin1 ==
  Clock : Clock
  sin_amplitude : Constant  Value=1.000000
  sin_bias : Constant  Value=0.000000
  sin_fcn : MATLAB Function  TreatAsAtomicUnit=on
  sin_frequency : Constant  Value=0.500000
  start_step_time : Constant  Value=10
  step_time_final : Constant  Value=10.000000
  sin : Outport  VectorParamsAs1DForOutWhenUnconnected=off
  wires:
  Clock/1 -> sin_fcn/4(time)
  sin_bias/1 -> sin_fcn/3(bias)
  sin_frequency/1 -> sin_fcn/2(frequency)
  sin_fcn/1(y) -> sin/1
  sin_amplitude/1 -> sin_fcn/1(amplitude)
  step_time_final/1 -> sin_fcn/6(end_time)
  start_step_time/1 -> sin_fcn/5(start_time)

== system Modele_LQR_3DOF/Subsystem/Simulation/p_sin2 ==
  Clock : Clock
  sin_amplitude : Constant  Value=1.000000
  sin_bias : Constant  Value=0.000000
  sin_fcn : MATLAB Function  TreatAsAtomicUnit=on
  sin_frequency : Constant  Value=0.500000
  start_step_time : Constant  Value=10
  step_time_final : Constant  Value=10.000000
  sin : Outport  VectorParamsAs1DForOutWhenUnconnected=off
  wires:
  Clock/1 -> sin_fcn/4(time)
  sin_bias/1 -> sin_fcn/3(bias)
  sin_frequency/1 -> sin_fcn/2(frequency)
  sin_fcn/1(y) -> sin/1
  sin_amplitude/1 -> sin_fcn/1(amplitude)
  step_time_final/1 -> sin_fcn/6(end_time)
  start_step_time/1 -> sin_fcn/5(start_time)

== system Modele_LQR_3DOF/Subsystem/Simulation/p_sin3 ==
  Clock : Clock
  sin_amplitude : Constant  Value=1.000000
  sin_bias : Constant  Value=0.000000
  sin_fcn : MATLAB Function  TreatAsAtomicUnit=on
  sin_frequency : Constant  Value=0.5
  start_step_time : Constant  Value=10
  step_time_final : Constant  Value=10.000000
  sin : Outport  VectorParamsAs1DForOutWhenUnconnected=off
  wires:
  Clock/1 -> sin_fcn/4(time)
  sin_bias/1 -> sin_fcn/3(bias)
  sin_frequency/1 -> sin_fcn/2(frequency)
  sin_fcn/1(y) -> sin/1
  sin_amplitude/1 -> sin_fcn/1(amplitude)
  step_time_final/1 -> sin_fcn/6(end_time)
  start_step_time/1 -> sin_fcn/5(start_time)

== system Modele_LQR_3DOF/Subsystem/Simulation/p_sin4 ==
  Clock : Clock
  sin_amplitude : Constant  Value=1.000000
  sin_bias : Constant  Value=0.000000
  sin_fcn : MATLAB Function  TreatAsAtomicUnit=on
  sin_frequency : Constant  Value=0.500000
  start_step_time : Constant  Value=3.000000
  step_time_final : Constant  Value=10.000000
  sin : Outport  VectorParamsAs1DForOutWhenUnconnected=off
  wires:
  Clock/1 -> sin_fcn/4(time)
  sin_bias/1 -> sin_fcn/3(bias)
  sin_frequency/1 -> sin_fcn/2(frequency)
  sin_fcn/1(y) -> sin/1
  sin_amplitude/1 -> sin_fcn/1(amplitude)
  step_time_final/1 -> sin_fcn/6(end_time)
  start_step_time/1 -> sin_fcn/5(start_time)

== system Modele_LQR_3DOF/Subsystem/Simulation/p_sin5 ==
  Clock : Clock
  sin_amplitude : Constant  Value=1.000000
  sin_bias : Constant  Value=0.000000
  sin_fcn : MATLAB Function  TreatAsAtomicUnit=on
  sin_frequency : Constant  Value=0.500000
  start_step_time : Constant  Value=3.000000
  step_time_final : Constant  Value=10.000000
  sin : Outport  VectorParamsAs1DForOutWhenUnconnected=off
  wires:
  Clock/1 -> sin_fcn/4(time)
  sin_bias/1 -> sin_fcn/3(bias)
  sin_frequency/1 -> sin_fcn/2(frequency)
  sin_fcn/1(y) -> sin/1
  sin_amplitude/1 -> sin_fcn/1(amplitude)
  step_time_final/1 -> sin_fcn/6(end_time)
  start_step_time/1 -> sin_fcn/5(start_time)

== system Modele_LQR_3DOF/Subsystem/Simulation/p_sin6 ==
  Clock : Clock
  sin_amplitude : Constant  Value=1.000000
  sin_bias : Constant  Value=0.000000
  sin_fcn : MATLAB Function  TreatAsAtomicUnit=on
  sin_frequency : Constant  Value=0.500000
  start_step_time : Constant  Value=3.000000
  step_time_final : Constant  Value=10.000000
  sin : Outport  VectorParamsAs1DForOutWhenUnconnected=off
  wires:
  Clock/1 -> sin_fcn/4(time)
  sin_bias/1 -> sin_fcn/3(bias)
  sin_frequency/1 -> sin_fcn/2(frequency)
  sin_fcn/1(y) -> sin/1
  sin_amplitude/1 -> sin_fcn/1(amplitude)
  step_time_final/1 -> sin_fcn/6(end_time)
  start_step_time/1 -> sin_fcn/5(start_time)

== system Modele_LQR_3DOF/Subsystem/Simulation/p_sin7 ==
  Clock : Clock
  sin_amplitude : Constant  Value=1.000000
  sin_bias : Constant  Value=0.000000
  sin_fcn : MATLAB Function  TreatAsAtomicUnit=on
  sin_frequency : Constant  Value=0.500000
  start_step_time : Constant  Value=3.000000
  step_time_final : Constant  Value=10.000000
  sin : Outport  VectorParamsAs1DForOutWhenUnconnected=off
  wires:
  Clock/1 -> sin_fcn/4(time)
  sin_bias/1 -> sin_fcn/3(bias)
  sin_frequency/1 -> sin_fcn/2(frequency)
  sin_fcn/1(y) -> sin/1
  sin_amplitude/1 -> sin_fcn/1(amplitude)
  step_time_final/1 -> sin_fcn/6(end_time)
  start_step_time/1 -> sin_fcn/5(start_time)

== system Modele_LQR_3DOF/Subsystem/Simulation/p_step1 ==
  Clock : Clock
  final_value : Constant  Value=1.000000
  initial_value : Constant  Value=0.000000
  start_step_time : Constant  Value=10
  step_fcn : MATLAB Function  TreatAsAtomicUnit=on
  step_time_final : Constant  Value=17
  v_scaling : Constant  Value=1.500000
  step : Outport  VectorParamsAs1DForOutWhenUnconnected=off
  wires:
  Clock/1 -> step_fcn/3(t)
  final_value/1 -> step_fcn/2(qf)
  step_fcn/1(traj) -> step/1
  initial_value/1 -> step_fcn/1(q0)
  start_step_time/1 -> step_fcn/4(ts)
  step_time_final/1 -> step_fcn/5(tf)
  v_scaling/1 -> step_fcn/6(V_scaling)

== system Modele_LQR_3DOF/Subsystem/Simulation/p_step2 ==
  Clock : Clock
  final_value : Constant  Value=1.000000
  initial_value : Constant  Value=0.000000
  start_step_time : Constant  Value=10
  step_fcn : MATLAB Function  TreatAsAtomicUnit=on
  step_time_final : Constant  Value=17
  v_scaling : Constant  Value=1.500000
  step : Outport  VectorParamsAs1DForOutWhenUnconnected=off
  wires:
  Clock/1 -> step_fcn/3(t)
  final_value/1 -> step_fcn/2(qf)
  step_fcn/1(traj) -> step/1
  initial_value/1 -> step_fcn/1(q0)
  start_step_time/1 -> step_fcn/4(ts)
  step_time_final/1 -> step_fcn/5(tf)
  v_scaling/1 -> step_fcn/6(V_scaling)

== system Modele_LQR_3DOF/Subsystem/Simulation/p_step3 ==
  Clock : Clock
  final_value : Constant  Value=3
  initial_value : Constant  Value=0
  start_step_time : Constant  Value=0
  step_fcn : MATLAB Function  TreatAsAtomicUnit=on
  step_time_final : Constant  Value=4
  v_scaling : Constant  Value=1.500000
  step : Outport  VectorParamsAs1DForOutWhenUnconnected=off
  wires:
  Clock/1 -> step_fcn/3(t)
  final_value/1 -> step_fcn/2(qf)
  step_fcn/1(traj) -> step/1
  initial_value/1 -> step_fcn/1(q0)
  start_step_time/1 -> step_fcn/4(ts)
  step_time_final/1 -> step_fcn/5(tf)
  v_scaling/1 -> step_fcn/6(V_scaling)

== system Modele_LQR_3DOF/Subsystem/Simulation/p_step4 ==
  Clock : Clock
  final_value : Constant  Value=1.5
  initial_value : Constant  Value=0.000000
  start_step_time : Constant
  step_fcn : MATLAB Function  TreatAsAtomicUnit=on
  step_time_final : Constant  Value=20
  v_scaling : Constant  Value=1.500000
  step : Outport  VectorParamsAs1DForOutWhenUnconnected=off
  wires:
  Clock/1 -> step_fcn/3(t)
  final_value/1 -> step_fcn/2(qf)
  step_fcn/1(traj) -> step/1
  initial_value/1 -> step_fcn/1(q0)
  start_step_time/1 -> step_fcn/4(ts)
  step_time_final/1 -> step_fcn/5(tf)
  v_scaling/1 -> step_fcn/6(V_scaling)

== system Modele_LQR_3DOF/Subsystem/Simulation/p_step5 ==
  Clock : Clock
  final_value : Constant  Value=1.000000
  initial_value : Constant  Value=0.000000
  start_step_time : Constant  Value=5
  step_fcn : MATLAB Function  TreatAsAtomicUnit=on
  step_time_final : Constant  Value=20
  v_scaling : Constant  Value=1.500000
  step : Outport  VectorParamsAs1DForOutWhenUnconnected=off
  wires:
  Clock/1 -> step_fcn/3(t)
  final_value/1 -> step_fcn/2(qf)
  step_fcn/1(traj) -> step/1
  initial_value/1 -> step_fcn/1(q0)
  start_step_time/1 -> step_fcn/4(ts)
  step_time_final/1 -> step_fcn/5(tf)
  v_scaling/1 -> step_fcn/6(V_scaling)

== system Modele_LQR_3DOF/Subsystem/Simulation/p_step6 ==
  Clock : Clock
  final_value : Constant  Value=1.000000
  initial_value : Constant  Value=0.000000
  start_step_time : Constant  Value=10
  step_fcn : MATLAB Function  TreatAsAtomicUnit=on
  step_time_final : Constant  Value=17
  v_scaling : Constant  Value=1.500000
  step : Outport  VectorParamsAs1DForOutWhenUnconnected=off
  wires:
  Clock/1 -> step_fcn/3(t)
  final_value/1 -> step_fcn/2(qf)
  step_fcn/1(traj) -> step/1
  initial_value/1 -> step_fcn/1(q0)
  start_step_time/1 -> step_fcn/4(ts)
  step_time_final/1 -> step_fcn/5(tf)
  v_scaling/1 -> step_fcn/6(V_scaling)

== system Modele_LQR_3DOF/Subsystem/Simulation/p_step7 ==
  Clock : Clock
  final_value : Constant  Value=1.000000
  initial_value : Constant  Value=0.000000
  start_step_time : Constant  Value=10
  step_fcn : MATLAB Function  TreatAsAtomicUnit=on
  step_time_final : Constant  Value=17
  v_scaling : Constant  Value=1.500000
  step : Outport  VectorParamsAs1DForOutWhenUnconnected=off
  wires:
  Clock/1 -> step_fcn/3(t)
  final_value/1 -> step_fcn/2(qf)
  step_fcn/1(traj) -> step/1
  initial_value/1 -> step_fcn/1(q0)
  start_step_time/1 -> step_fcn/4(ts)
  step_time_final/1 -> step_fcn/5(tf)
  v_scaling/1 -> step_fcn/6(V_scaling)

== matlab function Modele_LQR_3DOF/Subsystem/Simulation/p_sin1/sin_fcn ==
  data: amplitude input; y output; frequency input; bias input; time input; start_time input; end_time input
function y = fcn(amplitude, frequency, bias, time, start_time, end_time)
%#codegen
if ( time < start_time)
    y = bias;
elseif ( start_time <= time & time <= end_time + start_time) 
    y = amplitude*sin(2*pi*frequency*(time-start_time)) + bias;
else
    y = amplitude*sin(2*pi*frequency*(end_time+start_time)) + bias;
end

end

== matlab function Modele_LQR_3DOF/Subsystem/Simulation/p_sin3/sin_fcn ==
  data: amplitude input; y output; frequency input; bias input; time input; start_time input; end_time input
function y = fcn(amplitude, frequency, bias, time, start_time, end_time)
%#codegen
if ( time < start_time)
    y = bias;
elseif ( start_time <= time & time <= end_time + start_time) 
    y = amplitude*sin(2*pi*frequency*(time-start_time)) + bias;
else
    y = amplitude*sin(2*pi*frequency*(end_time+start_time)) + bias;
end

end
